simulink model "TimeStateControl_model"  (R2015a)
settings: Solver=ode45  StartTime=0.0  StopTime=10  RelTol=1e-3
values from neighbouring files (symbols this model uses):
  CurveConstant = CatmullRomSpline_Const    [TimeStateControl_config.m]
  delta_max = + pi / 9    (= 0.349065850399)    [TimeStateControl_config.m]
  delta_min = - pi / 9    (= -0.349065850399)    [TimeStateControl_config.m]
  InitialState = [ 4;8;pi/2 ]    [TimeStateControl_config.m]
  l = 0.256    [TimeStateControl_config.m]
  NumOfCriteria = 4    [TimeStateControl_config.m]
  NumOfSection = length( x_vector ) - ( NumOfCriteria - 1 )    [TimeStateControl_config.m]
  x_vector = [  1,  3,  6,  7,  9, 11,  13 ]    [TimeStateControl_config.m]
  y_vector = [  4,  7,  6,  3,  1,  3,  7 ]    [TimeStateControl_config.m]
settings Model: Creator=hamada  LastModifiedBy=hamada

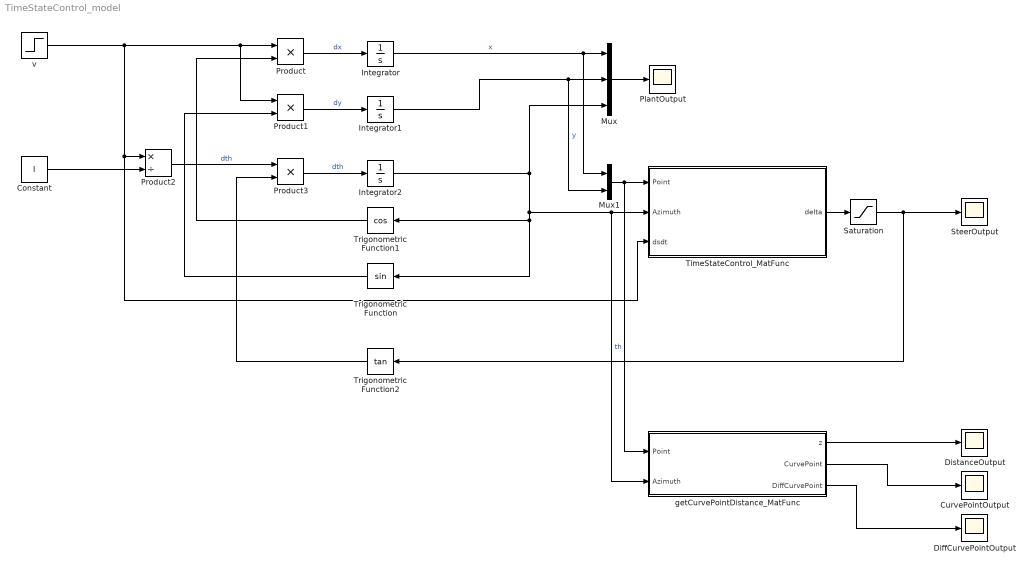
== system TimeStateControl_model ==
  Constant : Constant  Value=l
  CurvePointOutput : Scope
      settings: YMin=-0.25  YMax=1.5  SaveName=CurvePointOutput  SampleInput=on  SampleTime=SimPeriod
  DiffCurvePointOutput : Scope
      settings: YMin=-0.25  YMax=1.5  SaveName=DiffCurvePointOutput  SampleInput=on  SampleTime=SimPeriod
  DistanceOutput : Scope
      settings: YMin=-0.25  YMax=1.5  SaveName=DistanceOutput  SampleInput=on  SampleTime=SimPeriod
  Integrator : Integrator  InitialCondition=InitialState(1)
  Integrator1 : Integrator  InitialCondition=InitialState(2)
  Integrator2 : Integrator  InitialCondition=InitialState(3)
  Mux : Mux  Inputs=3
  Mux1 : Mux  Inputs=2
  PlantOutput : Scope
      settings: SaveName=PlantOutput  SampleInput=on  SampleTime=SimPeriod
  Product : Product
  Product1 : Product
  Product2 : Product  Inputs=*/
  Product3 : Product
  Saturation : Saturate  UpperLimit=delta_max  LowerLimit=delta_min
  SteerOutput : Scope
      settings: TimeRange=30  SaveName=SteerOutput  SampleInput=on  SampleTime=SimPeriod
  TimeStateControl_MatFunc : MATLAB Function  TreatAsAtomicUnit=on
  Trigonometric Function : Trigonometry
  Trigonometric Function1 : Trigonometry  Operator=cos
  Trigonometric Function2 : Trigonometry  Operator=tan
  getCurvePointDistance_MatFunc : MATLAB Function  TreatAsAtomicUnit=on
  v : Step  Time=5  Before=0.3  After=0.3  SampleTime=0
  wires:
  Product1/1 -> Integrator1/1  "dy"
  Product/1 -> Integrator/1  "dx"
  Product3/1 -> Integrator2/1  "dth"
  Integrator2/1 -> Mux/3, Trigonometric Function/1, Trigonometric Function1/1, getCurvePointDistance_MatFunc/2(Azimuth), TimeStateControl_MatFunc/2(Azimuth)  "th"
  Integrator1/1 -> Mux1/2, Mux/2  "y"
  Integrator/1 -> Mux1/1, Mux/1  "x"
  Trigonometric Function1/1 -> Product/2
  v/1 -> TimeStateControl_MatFunc/3(dsdt), Product2/1, Product1/1, Product/1
  Trigonometric Function/1 -> Product1/2
  Saturation/1 -> Trigonometric Function2/1, SteerOutput/1
  Constant/1 -> Product2/2
  Mux/1 -> PlantOutput/1
  Mux1/1 -> TimeStateControl_MatFunc/1(Point), getCurvePointDistance_MatFunc/1(Point)
  TimeStateControl_MatFunc/1(delta) -> Saturation/1
  Product2/1 -> Product3/1  "dth"
  Trigonometric Function2/1 -> Product3/2
  getCurvePointDistance_MatFunc/1(z) -> DistanceOutput/1
  getCurvePointDistance_MatFunc/2(CurvePoint) -> CurvePointOutput/1
  getCurvePointDistance_MatFunc/3(DiffCurvePoint) -> DiffCurvePointOutput/1

== matlab function TimeStateControl_model/getCurvePointDistance_MatFunc ==
  settings: updateMethod=DISCRETE  sampleTime=SamplingPeriod
  data: Point input size=2; Azimuth input; z output; x_vector parameter; y_vector parameter; l parameter size=1; NumOfSection parameter size=1; NumOfCriteria parameter size=1; CurveConstant parameter size=4,4; CurvePoint output; DiffCurvePoint output
function [ z, CurvePoint, DiffCurvePoint ] = getCurvePointDistance_MatFunc( Point, Azimuth, x_vector, y_vector, l, NumOfSection, NumOfCriteria, CurveConstant )
    [ section_min, t_min ] = getNearestCurveParameter_AllSection( Point, x_vector, y_vector, NumOfSection, NumOfCriteria, CurveConstant );
    
    Criteria = [ 
        x_vector(section_min:section_min+(NumOfCriteria-1));
        y_vector(section_min:section_min+(NumOfCriteria-1));
    ];

    CurvePoint = getCurvePoint( t_min, Criteria, CurveConstant );
    DiffCurvePoint = getDiffCurvePoint( t_min, Criteria, CurveConstant );
    DiffCurvePoint = DiffCurvePoint / norm( DiffCurvePoint );

    z = getCurvePointDistance( Point, CurvePoint ) * getCurvePointSide( Point, CurvePoint, DiffCurvePoint );
    
end

== matlab function TimeStateControl_model/TimeStateControl_MatFunc ==
  settings: updateMethod=DISCRETE  sampleTime=SamplingPeriod
  data: Point input size=2; Azimuth input; dsdt input; delta output; x_vector parameter; y_vector parameter; l parameter size=1; NumOfSection parameter size=1; NumOfCriteria parameter size=1; CurveConstant parameter size=4,4
function delta = TimeStateControl_MatFunc( Point, Azimuth, dsdt, x_vector, y_vector, l, NumOfSection, NumOfCriteria, CurveConstant )
    delta = TimeStateControl( Point, Azimuth, dsdt, x_vector, y_vector, l, NumOfSection, NumOfCriteria, CurveConstant );
end
